simulink library "power_quality_lib"  (Simulink 8.1)
settings: Solver=ode45  StartTime=0.0  StopTime=10.0  RelTol=1e-3
undefined symbols (not defined in the file): DiscIntNeverNeededParam, Ts
settings Model: Creator=re25624  LastModifiedBy=hptb1

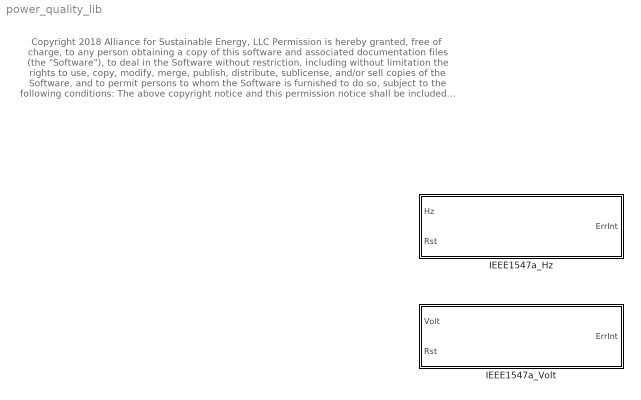
== system power_quality_lib ==
  note: Copyright 2018 Alliance for Sustainable Energy, LLC
      |
      | Permission is hereby granted, free of charge, to any person obtaining a copy of this software
      | and associated documentation files (the "Software"), to deal in the Software without restriction,
      | including without limitation the rights to use, copy, modify, merge, publish, distribute, sublicense,
      | and/or sell copies of the Software, and to permit persons to whom the Software is furnished to do so,
      | subject to the following conditions:
      |
      | The above copyright notice and this permission notice shall be included in all copies or substantial portions of the Software.
      |
      | THE SOFTWARE IS PROVIDED "AS IS", WITHOUT WARRANTY OF ANY KIND, EXPRESS OR IMPLIED, INCLUDING
      | BUT NOT LIMITED TO THE WARRANTIES OF MERCHANTABILITY, FITNESS FOR A PARTICULAR PURPOSE AND
      | NONINFRINGEMENT. IN NO EVENT SHALL THE AUTHORS, THE COPYRIGHT HOLDERS, THE UNITED STATES,
      | THE UNITED STATES DEPARTMENT OF ENERGY, OR ANY OF THEIR EMPLOYEES BE LIABLE FOR ANY CLAIM,
      | DAMAGES OR OTHER LIABILITY, WHETHER IN AN ACTION OF CONTRACT, TORT OR OTHERWISE, ARISING FROM,
      | OUT OF OR IN CONNECTION WITH THE SOFTWARE OR THE USE OR OTHER DEALINGS IN THE SOFTWARE.
  IEEE1547a_Hz : Subsystem
  IEEE1547a_Volt : Subsystem

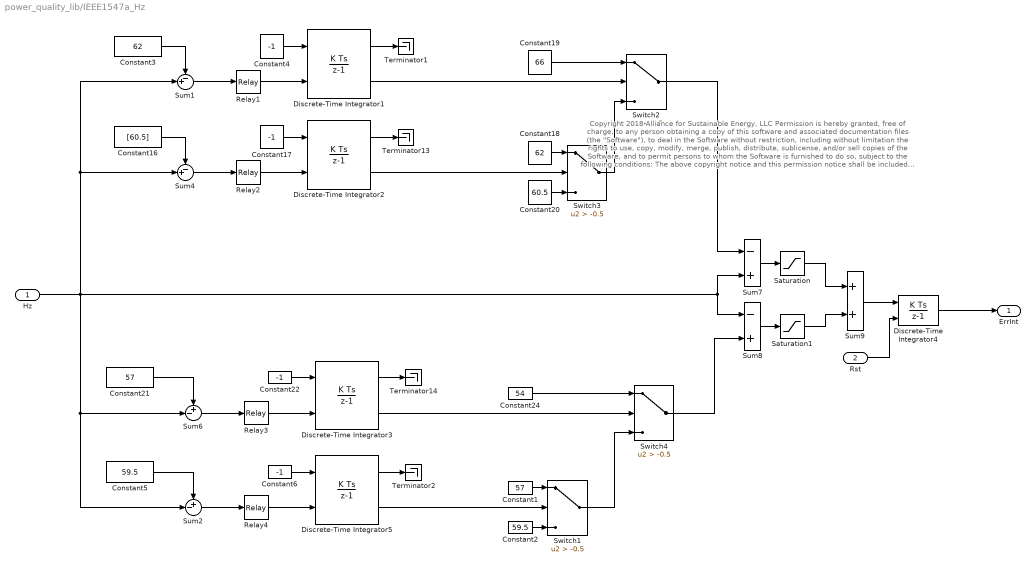
== system power_quality_lib/IEEE1547a_Hz ==
  note: Copyright 2018 Alliance for Sustainable Energy, LLC
      |
      | Permission is hereby granted, free of charge, to any person obtaining a copy of this software
      | and associated documentation files (the "Software"), to deal in the Software without restriction,
      | including without limitation the rights to use, copy, modify, merge, publish, distribute, sublicense,
      | and/or sell copies of the Software, and to permit persons to whom the Software is furnished to do so,
      | subject to the following conditions:
      |
      | The above copyright notice and this permission notice shall be included in all copies or substantial portions of the Software.
      |
      | THE SOFTWARE IS PROVIDED "AS IS", WITHOUT WARRANTY OF ANY KIND, EXPRESS OR IMPLIED, INCLUDING
      | BUT NOT LIMITED TO THE WARRANTIES OF MERCHANTABILITY, FITNESS FOR A PARTICULAR PURPOSE AND
      | NONINFRINGEMENT. IN NO EVENT SHALL THE AUTHORS, THE COPYRIGHT HOLDERS, THE UNITED STATES,
      | THE UNITED STATES DEPARTMENT OF ENERGY, OR ANY OF THEIR EMPLOYEES BE LIABLE FOR ANY CLAIM,
      | DAMAGES OR OTHER LIABILITY, WHETHER IN AN ACTION OF CONTRACT, TORT OR OTHERWISE, ARISING FROM,
      | OUT OF OR IN CONNECTION WITH THE SOFTWARE OR THE USE OR OTHER DEALINGS IN THE SOFTWARE.
  Hz : Inport
  Rst : Inport  Port=2
  Constant1 : Constant  Value=57
  Constant16 : Constant  Value=[60.5]
  Constant{4,6,17,22} (4 alike) : Constant  Value=-1
  Constant18 : Constant  Value=62
  Constant19 : Constant  Value=66
  Constant2 : Constant  Value=59.5
  Constant20 : Constant  Value=60.5
  Constant21 : Constant  Value=57
  Constant24 : Constant  Value=54
  Constant3 : Constant  Value=62
  Constant5 : Constant  Value=59.5
  Discrete-Time Integrator1 : DiscreteIntegrator  gainval=1  ExternalReset=rising  InitialCondition=0.16  SampleTime=Ts  LimitOutput=on  LowerSaturationLimit=0  ShowSaturationPort=on  ICPrevOutput=DiscIntNeverNeededParam  ICPrevScaledInput=DiscIntNeverNeededParam
  Discrete-Time Integrator2 : DiscreteIntegrator  gainval=1  ExternalReset=rising  InitialCondition=2  SampleTime=Ts  LimitOutput=on  LowerSaturationLimit=0  ShowSaturationPort=on  ICPrevOutput=DiscIntNeverNeededParam  ICPrevScaledInput=DiscIntNeverNeededParam
  Discrete-Time Integrator3 : DiscreteIntegrator  gainval=1  ExternalReset=rising  InitialCondition=0.16  SampleTime=Ts  LimitOutput=on  LowerSaturationLimit=0  ShowSaturationPort=on  ICPrevOutput=DiscIntNeverNeededParam  ICPrevScaledInput=DiscIntNeverNeededParam
  Discrete-Time Integrator4 : DiscreteIntegrator  gainval=1  ExternalReset=level  SampleTime=Ts  LowerSaturationLimit=0  ICPrevOutput=DiscIntNeverNeededParam  ICPrevScaledInput=DiscIntNeverNeededParam
  Discrete-Time Integrator5 : DiscreteIntegrator  gainval=1  ExternalReset=rising  InitialCondition=2  SampleTime=Ts  LimitOutput=on  LowerSaturationLimit=0  ShowSaturationPort=on  ICPrevOutput=DiscIntNeverNeededParam  ICPrevScaledInput=DiscIntNeverNeededParam
  Relay{1..4} (4 alike) : Relay  OnSwitchValue=0.02  OffSwitchValue=-0.02
  Saturation : Saturate  UpperLimit=6  LowerLimit=0
  Saturation1 : Saturate  UpperLimit=6  LowerLimit=0
  Sum1 : Sum  Inputs=-+|
  Sum2 : Sum  Inputs=+-|
  Sum4 : Sum  Inputs=-+|
  Sum6 : Sum  Inputs=+-|
  Sum7 : Sum  Inputs=-+
  Sum8 : Sum  Inputs=-+
  Sum9 : Sum
  Switch{1..4} (4 alike) : Switch  Criteria=u2 > Threshold  Threshold=-0.5
  Terminator{1..2,13..14} (4 alike) : Terminator
  ErrInt : Outport
  wires:
  Saturation/1 -> Sum9/1
  Saturation1/1 -> Sum9/2
  Hz/1 -> Sum2/2, Sum6/2, Sum4/2, Sum1/2, Sum8/1, Sum7/2
  Constant5/1 -> Sum2/1
  Sum2/1 -> Relay4/1
  Discrete-Time Integrator5/1 -> Terminator2/1
  Relay4/1 -> Discrete-Time Integrator5/2
  Constant6/1 -> Discrete-Time Integrator5/1
  Constant3/1 -> Sum1/1
  Sum1/1 -> Relay1/1
  Relay1/1 -> Discrete-Time Integrator1/2
  Discrete-Time Integrator1/1 -> Terminator1/1
  Constant4/1 -> Discrete-Time Integrator1/1
  Discrete-Time Integrator5/2 -> Switch1/2
  Constant2/1 -> Switch1/3
  Constant1/1 -> Switch1/1
  Constant21/1 -> Sum6/1
  Sum6/1 -> Relay3/1
  Discrete-Time Integrator3/2 -> Switch4/2
  Discrete-Time Integrator3/1 -> Terminator14/1
  Relay3/1 -> Discrete-Time Integrator3/2
  Constant24/1 -> Switch4/1
  Constant22/1 -> Discrete-Time Integrator3/1
  Switch1/1 -> Switch4/3
  Constant19/1 -> Switch2/1
  Constant18/1 -> Switch3/1
  Switch3/1 -> Switch2/3
  Discrete-Time Integrator1/2 -> Switch2/2
  Discrete-Time Integrator2/2 -> Switch3/2
  Constant20/1 -> Switch3/3
  Discrete-Time Integrator4/1 -> ErrInt/1
  Sum8/1 -> Saturation1/1
  Rst/1 -> Discrete-Time Integrator4/2
  Sum7/1 -> Saturation/1
  Switch4/1 -> Sum8/2
  Switch2/1 -> Sum7/1
  Sum9/1 -> Discrete-Time Integrator4/1
  Constant16/1 -> Sum4/1
  Sum4/1 -> Relay2/1
  Relay2/1 -> Discrete-Time Integrator2/2
  Discrete-Time Integrator2/1 -> Terminator13/1
  Constant17/1 -> Discrete-Time Integrator2/1

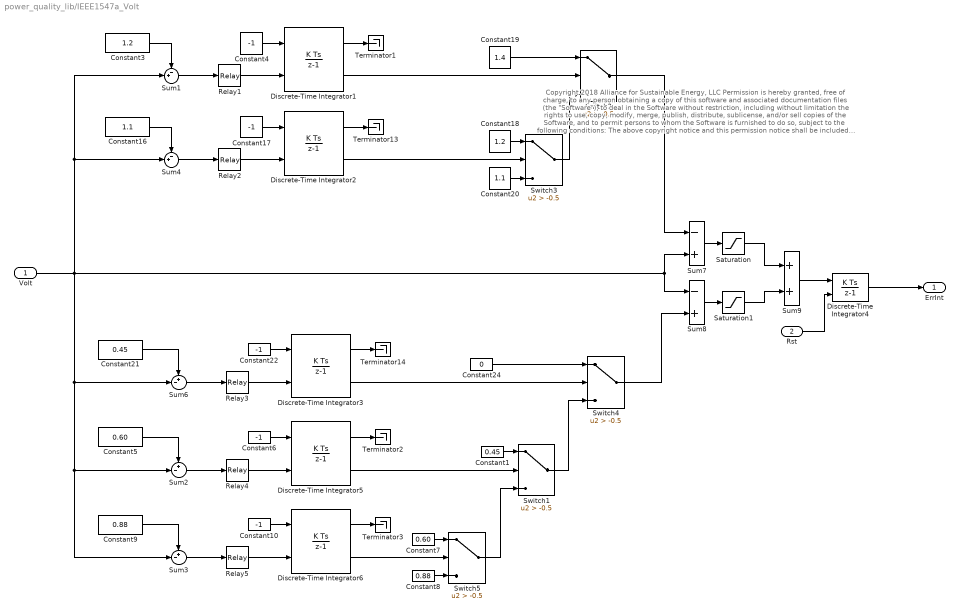
== system power_quality_lib/IEEE1547a_Volt ==
  note: Copyright 2018 Alliance for Sustainable Energy, LLC
      |
      | Permission is hereby granted, free of charge, to any person obtaining a copy of this software
      | and associated documentation files (the "Software"), to deal in the Software without restriction,
      | including without limitation the rights to use, copy, modify, merge, publish, distribute, sublicense,
      | and/or sell copies of the Software, and to permit persons to whom the Software is furnished to do so,
      | subject to the following conditions:
      |
      | The above copyright notice and this permission notice shall be included in all copies or substantial portions of the Software.
      |
      | THE SOFTWARE IS PROVIDED "AS IS", WITHOUT WARRANTY OF ANY KIND, EXPRESS OR IMPLIED, INCLUDING
      | BUT NOT LIMITED TO THE WARRANTIES OF MERCHANTABILITY, FITNESS FOR A PARTICULAR PURPOSE AND
      | NONINFRINGEMENT. IN NO EVENT SHALL THE AUTHORS, THE COPYRIGHT HOLDERS, THE UNITED STATES,
      | THE UNITED STATES DEPARTMENT OF ENERGY, OR ANY OF THEIR EMPLOYEES BE LIABLE FOR ANY CLAIM,
      | DAMAGES OR OTHER LIABILITY, WHETHER IN AN ACTION OF CONTRACT, TORT OR OTHERWISE, ARISING FROM,
      | OUT OF OR IN CONNECTION WITH THE SOFTWARE OR THE USE OR OTHER DEALINGS IN THE SOFTWARE.
  Volt : Inport
  Rst : Inport  Port=2
  Constant1 : Constant  Value=0.45
  Constant{4,6,10,17,22} (5 alike) : Constant  Value=-1
  Constant16 : Constant  Value=1.1
  Constant18 : Constant  Value=1.2
  Constant19 : Constant  Value=1.4
  Constant20 : Constant  Value=1.1
  Constant21 : Constant  Value=0.45
  Constant24 : Constant  Value=0
  Constant3 : Constant  Value=1.2
  Constant5 : Constant  Value=0.60
  Constant7 : Constant  Value=0.60
  Constant8 : Constant  Value=0.88
  Constant9 : Constant  Value=0.88
  Discrete-Time Integrator1 : DiscreteIntegrator  gainval=1  ExternalReset=rising  InitialCondition=0.16  SampleTime=Ts  LimitOutput=on  LowerSaturationLimit=0  ShowSaturationPort=on  ICPrevOutput=DiscIntNeverNeededParam  ICPrevScaledInput=DiscIntNeverNeededParam
  Discrete-Time Integrator2 : DiscreteIntegrator  gainval=1  ExternalReset=rising  InitialCondition=1  SampleTime=Ts  LimitOutput=on  LowerSaturationLimit=0  ShowSaturationPort=on  ICPrevOutput=DiscIntNeverNeededParam  ICPrevScaledInput=DiscIntNeverNeededParam
  Discrete-Time Integrator3 : DiscreteIntegrator  gainval=1  ExternalReset=rising  InitialCondition=0.16  SampleTime=Ts  LimitOutput=on  LowerSaturationLimit=0  ShowSaturationPort=on  ICPrevOutput=DiscIntNeverNeededParam  ICPrevScaledInput=DiscIntNeverNeededParam
  Discrete-Time Integrator4 : DiscreteIntegrator  gainval=1  ExternalReset=level  SampleTime=Ts  LowerSaturationLimit=0  ICPrevOutput=DiscIntNeverNeededParam  ICPrevScaledInput=DiscIntNeverNeededParam
  Discrete-Time Integrator5 : DiscreteIntegrator  gainval=1  ExternalReset=rising  InitialCondition=1  SampleTime=Ts  LimitOutput=on  LowerSaturationLimit=0  ShowSaturationPort=on  ICPrevOutput=DiscIntNeverNeededParam  ICPrevScaledInput=DiscIntNeverNeededParam
  Discrete-Time Integrator6 : DiscreteIntegrator  gainval=1  ExternalReset=rising  InitialCondition=2  SampleTime=Ts  LimitOutput=on  LowerSaturationLimit=0  ShowSaturationPort=on  ICPrevOutput=DiscIntNeverNeededParam  ICPrevScaledInput=DiscIntNeverNeededParam
  Relay{1..5} (5 alike) : Relay  OnSwitchValue=0.02  OffSwitchValue=-0.02
  Saturation : Saturate  UpperLimit=6  LowerLimit=0
  Saturation1 : Saturate  UpperLimit=6  LowerLimit=0
  Sum1 : Sum  Inputs=-+|
  Sum2 : Sum  Inputs=+-|
  Sum3 : Sum  Inputs=+-|
  Sum4 : Sum  Inputs=-+|
  Sum6 : Sum  Inputs=+-|
  Sum7 : Sum  Inputs=-+
  Sum8 : Sum  Inputs=-+
  Sum9 : Sum
  Switch{1..5} (5 alike) : Switch  Criteria=u2 > Threshold  Threshold=-0.5
  Terminator{1..3,13..14} (5 alike) : Terminator
  ErrInt : Outport
  wires:
  Constant17/1 -> Discrete-Time Integrator2/1
  Discrete-Time Integrator2/1 -> Terminator13/1
  Relay2/1 -> Discrete-Time Integrator2/2
  Sum4/1 -> Relay2/1
  Constant16/1 -> Sum4/1
  Sum9/1 -> Discrete-Time Integrator4/1
  Switch2/1 -> Sum7/1
  Switch4/1 -> Sum8/2
  Sum7/1 -> Saturation/1
  Rst/1 -> Discrete-Time Integrator4/2
  Sum8/1 -> Saturation1/1
  Discrete-Time Integrator4/1 -> ErrInt/1
  Constant20/1 -> Switch3/3
  Discrete-Time Integrator2/2 -> Switch3/2
  Discrete-Time Integrator1/2 -> Switch2/2
  Switch3/1 -> Switch2/3
  Constant18/1 -> Switch3/1
  Constant19/1 -> Switch2/1
  Switch1/1 -> Switch4/3
  Constant22/1 -> Discrete-Time Integrator3/1
  Constant24/1 -> Switch4/1
  Relay3/1 -> Discrete-Time Integrator3/2
  Discrete-Time Integrator3/1 -> Terminator14/1
  Discrete-Time Integrator3/2 -> Switch4/2
  Sum6/1 -> Relay3/1
  Constant21/1 -> Sum6/1
  Constant1/1 -> Switch1/1
  Switch5/1 -> Switch1/3
  Discrete-Time Integrator5/2 -> Switch1/2
  Constant4/1 -> Discrete-Time Integrator1/1
  Discrete-Time Integrator1/1 -> Terminator1/1
  Relay1/1 -> Discrete-Time Integrator1/2
  Sum1/1 -> Relay1/1
  Constant3/1 -> Sum1/1
  Constant6/1 -> Discrete-Time Integrator5/1
  Relay4/1 -> Discrete-Time Integrator5/2
  Discrete-Time Integrator5/1 -> Terminator2/1
  Sum2/1 -> Relay4/1
  Constant5/1 -> Sum2/1
  Saturation1/1 -> Sum9/2
  Saturation/1 -> Sum9/1
  Constant7/1 -> Switch5/1
  Constant8/1 -> Switch5/3
  Discrete-Time Integrator6/2 -> Switch5/2
  Constant10/1 -> Discrete-Time Integrator6/1
  Relay5/1 -> Discrete-Time Integrator6/2
  Discrete-Time Integrator6/1 -> Terminator3/1
  Sum3/1 -> Relay5/1
  Constant9/1 -> Sum3/1
  Volt/1 -> Sum7/2, Sum8/1, Sum1/2, Sum4/2, Sum3/2, Sum2/2, Sum6/2
